simulink model "RL_TTS3_Controller_Blank"  (R2019b)
settings: Solver=FixedStepAuto  StartTime=0.0  StopTime=10.0  FixedStep=0.01  RelTol=1e-3
PostLoadFcn:
  | if any(exist('dsrtsu_mdlpostloadfcn', 'file') ~= 0), dsrtsu_mdlpostloadfcn('Execute', bdroot); end
values from neighbouring files (symbols this model uses):
  SetPumpR = 0    [RL_TTS3_Controller_Blank.mat]    (also in RL_TTS3_Controller_Blank_DefaultVal.mat)
  ValveLD_close = 0    [RL_TTS3_Controller_Blank.mat]    (also in RL_TTS3_Controller_Blank_DefaultVal.mat)
  ValveLD_open = 0    [RL_TTS3_Controller_Blank.mat]    (also in RL_TTS3_Controller_Blank_DefaultVal.mat)
  ValveLM_close = 0    [RL_TTS3_Controller_Blank.mat]    (also in RL_TTS3_Controller_Blank_DefaultVal.mat)
  ValveLM_open = 0    [RL_TTS3_Controller_Blank.mat]    (also in RL_TTS3_Controller_Blank_DefaultVal.mat)
  ValveMD_close = 0    [RL_TTS3_Controller_Blank.mat]    (also in RL_TTS3_Controller_Blank_DefaultVal.mat)
  ValveMD_open = 0    [RL_TTS3_Controller_Blank.mat]    (also in RL_TTS3_Controller_Blank_DefaultVal.mat)
  ValveMR_close = 0    [RL_TTS3_Controller_Blank.mat]    (also in RL_TTS3_Controller_Blank_DefaultVal.mat)
  ValveMR_open = 0    [RL_TTS3_Controller_Blank.mat]    (also in RL_TTS3_Controller_Blank_DefaultVal.mat)
  ValveRD_close = 0    [RL_TTS3_Controller_Blank.mat]    (also in RL_TTS3_Controller_Blank_DefaultVal.mat)
  ValveRD_open = 0    [RL_TTS3_Controller_Blank.mat]    (also in RL_TTS3_Controller_Blank_DefaultVal.mat)
libraries: simulink x1
settings Model: DSRTSU_INTERNAL_RTI_VER=550  DSRTSU_INTERNAL_RTI_TYPE=rti1104  RTICANMMDATA=struct('GeneralSetupData',struct('modelroot','E:\Will\RemoteLabs\TTS3\HostPC','generalsettings',struct('filesettings',struct('destfolder',struct('Name','RTICANMM_FILES','Check',1),'buildfolder',struct('Name','.','Check',1),'AbsDestfolder',struct('Name','E:\Will\RemoteLabs\TTS3\HostPC\RTICANMM_FILES'),'AbsBuildfolder',struct('Name','E:\Will\RemoteLabs\TTS3\HostPC'))),'options',struct('addpaths',1,'rmpaths',1,'addtrcexclusion',true,'cannavigator',struct('checkmonitoring',0),'show_usrtrc',0,'use_usrtrc',0),'advanced',struct('options',ones(1,100)),'MPSetup',{{}},'RTI',struct('Type','RTI1104','Ver','7.13','Date','02-Nov-2019'),'modelname','TTS3_Controller_Test_OL','block','TTS3_Controller_Test_OL'))  DSRTSU_INTERNAL_RTIFPGA=150  Creator=whendrix  LastModifiedBy=maxva
settings OptimizationCC: BlockReduction=off  OptimizeBlockIOStorage=off  BufferReuse=off  GlobalBufferReuse=off  ExpressionFolding=off  LocalBlockOutputs=off  OptimizeDataStoreBuffers=off  BusAssignmentInplaceUpdate=off
settings DebuggingCC: BusObjectLabelMismatch=none
settings HardwareCC: ProdBitPerPointer=32  ProdBitPerSizeT=32  ProdBitPerPtrDiffT=32  ProdLargestAtomicInteger=Integer  ProdEndianess=BigEndian  ProdWordSize=32  ProdHWDeviceType=Custom Processor->Custom  TargetIntDivRoundTo=Zero  TargetEndianess=BigEndian  TargetHWDeviceType=Custom Processor->Custom
settings ModelReferenceCC: ModelReferenceNumInstancesAllowed=Single  ModelReferenceMinAlgLoopOccurrences=on
settings SFSimCC: MATLABDynamicMemAlloc=off  CustomCodeUndefinedFunction=UseInterfaceOnly
settings RTWCC: Description=dSPACE DS1104 Hardware Platform  SystemTargetFile=rti1104.tlc  MakeCommand=make_rti  TemplateMakefile=rti1104.tmf
settings CodeAppCC: MaxIdLength=63
settings STFCustomTargetCC: ParMdlRefBuildCompliant=on  SystemTargetFile=rti1104.tlc
settings GRTTargetCC: TargetLangStandard=C89/C90 (ANSI)  CompOptLevelCompliant=off  ConcurrentExecutionCompliant=off  CombineOutputUpdateFcns=off  MatFileLogging=off  CPPClassGenCompliant=off  UseToolchainInfoCompliant=off

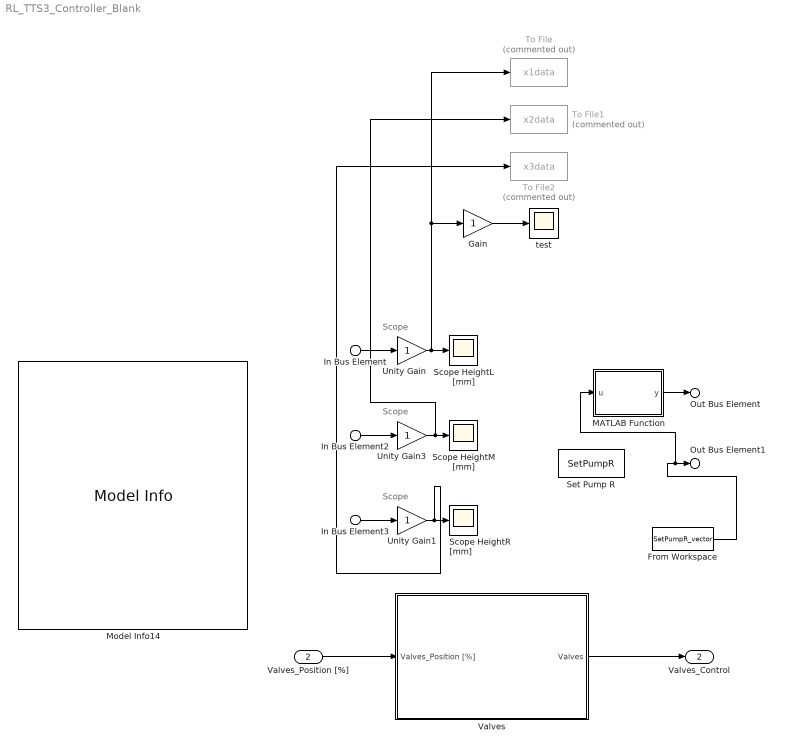
== system RL_TTS3_Controller_Blank ==
  note: Scope
  note: Scope
  note: Scope
  In Bus Element : Inport  PortName=Heights [mm]  Element=Left
  In Bus Element2 : Inport  PortName=Heights [mm]  Element=Middle
  In Bus Element3 : Inport  PortName=Heights [mm]  Element=Right
  Valves_Position [%] : Inport  Port=2  OutDataTypeStr=Bus: ValvesSOCI
  From Workspace : FromWorkspace  VariableName=SetPumpR_vector
  Gain : Gain
  MATLAB Function : MATLAB Function  TreatAsAtomicUnit=on
  Model Info14 : simulink/Model-Wide Utilities/Model Info  Frame=on  DisplayStringWithTags=|  HorizontalTextAlignment=Left  LeftAlignmentValue=0.02
      | Start model for the "Three Tank"
      | experiment on the "Three Tank" setup.
      | Version: 1.0
      | 
      | 
      | INFORMATION
      | ----------------------
      | 
      | Unity Gain block before Scope is needed for
      | RemoteLabs compatebility. 
      | Do not modify or remove!
      | 
      | Pump range:
      | 0 to 0.102 [l/s]
      | 
      | The 5 Valves are labeled according 
      | to their position:
      | 
      |    LM  MR
      |      X     X
      |  X      X      X
      | LD    MD   RD
      | 
      | L = Left
      | M = Middle
      | R = Right
      | D = Down
  Scope HeightL [mm] : Scope
  Scope HeightM [mm] : Scope
  Scope HeightR [mm] : Scope
  Set Pump R : Constant  Value=SetPumpR
  To File : ToFile  Commented=on  Filename=x1data  MatrixName=x1
  To File1 : ToFile  Commented=on  Filename=x2data  MatrixName=x2
  To File2 : ToFile  Commented=on  Filename=x3data  MatrixName=x3
  Unity Gain : Gain
  Unity Gain1 : Gain
  Unity Gain3 : Gain
  Valves : Subsystem  TreatAsAtomicUnit=on
  test : Scope
  Out Bus Element : Outport  VectorParamsAs1DForOutWhenUnconnected=off  PortName=Pumps [l/s]  Element=Left
  Out Bus Element1 : Outport  VectorParamsAs1DForOutWhenUnconnected=off  PortName=Pumps [l/s]  Element=Right
  Valves_Control : Outport  Port=2  OutDataTypeStr=Bus: ValvesSICO  VectorParamsAs1DForOutWhenUnconnected=off
  wires:
  Unity Gain3/1 -> To File1/1, Scope HeightM [mm]/1
  Unity Gain1/1 -> To File2/1, Scope HeightR [mm]/1
  In Bus Element/1 -> Unity Gain/1
  In Bus Element2/1 -> Unity Gain3/1
  In Bus Element3/1 -> Unity Gain1/1
  Valves/1(Valves) -> Valves_Control/1
  Valves_Position [%]/1 -> Valves/1(Valves_Position [%])
  Unity Gain/1 -> Gain/1, To File/1, Scope HeightL [mm]/1
  From Workspace/1 -> MATLAB Function/1(u), Out Bus Element1/1
  Gain/1 -> test/1
  MATLAB Function/1(y) -> Out Bus Element/1

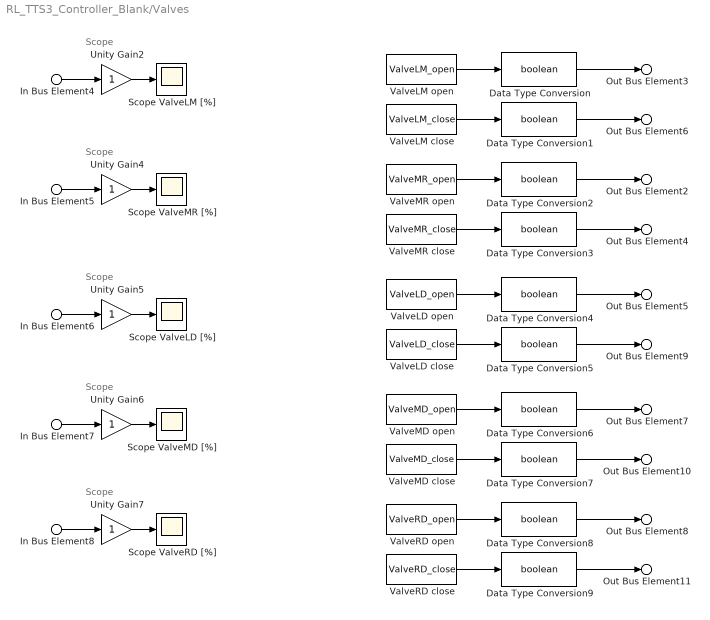
== system RL_TTS3_Controller_Blank/Valves ==
  note: Scope
  note: Scope
  note: Scope
  note: Scope
  note: Scope
  In Bus Element4 : Inport  PortName=Valves_Position [%]  Element=LeftMiddle
  In Bus Element5 : Inport  PortName=Valves_Position [%]  Element=MiddleRight
  In Bus Element6 : Inport  PortName=Valves_Position [%]  Element=LeftDown
  In Bus Element7 : Inport  PortName=Valves_Position [%]  Element=MiddleDown
  In Bus Element8 : Inport  PortName=Valves_Position [%]  Element=RightDown
  Data Type Conversion{,1..9} (10 alike) : DataTypeConversion  OutDataTypeStr=boolean
  Scope ValveLD [%] : Scope
  Scope ValveLM [%] : Scope
  Scope ValveMD [%] : Scope
  Scope ValveMR [%] : Scope
  Scope ValveRD [%] : Scope
  Unity Gain{2,4..7} (5 alike) : Gain
  ValveLD close : Constant  Value=ValveLD_close  OutDataTypeStr=double
  ValveLD open : Constant  Value=ValveLD_open  OutDataTypeStr=double
  ValveLM close : Constant  Value=ValveLM_close  OutDataTypeStr=double
  ValveLM open : Constant  Value=ValveLM_open  OutDataTypeStr=double
  ValveMD close : Constant  Value=ValveMD_close  OutDataTypeStr=double
  ValveMD open : Constant  Value=ValveMD_open  OutDataTypeStr=double
  ValveMR close : Constant  Value=ValveMR_close  OutDataTypeStr=double
  ValveMR open : Constant  Value=ValveMR_open  OutDataTypeStr=double
  ValveRD close : Constant  Value=ValveRD_close  OutDataTypeStr=double
  ValveRD open : Constant  Value=ValveRD_open  OutDataTypeStr=double
  Out Bus Element8 : Outport  VectorParamsAs1DForOutWhenUnconnected=off  PortName=Valves  Element=RightDown.Open
  Out Bus Element11 : Outport  VectorParamsAs1DForOutWhenUnconnected=off  PortName=Valves  Element=RightDown.Close
  Out Bus Element5 : Outport  VectorParamsAs1DForOutWhenUnconnected=off  PortName=Valves  Element=LeftDown.Open
  Out Bus Element9 : Outport  VectorParamsAs1DForOutWhenUnconnected=off  PortName=Valves  Element=LeftDown.Close
  Out Bus Element7 : Outport  VectorParamsAs1DForOutWhenUnconnected=off  PortName=Valves  Element=MiddleDown.Open
  Out Bus Element10 : Outport  VectorParamsAs1DForOutWhenUnconnected=off  PortName=Valves  Element=MiddleDown.Close
  Out Bus Element2 : Outport  VectorParamsAs1DForOutWhenUnconnected=off  PortName=Valves  Element=MiddleRight.Open
  Out Bus Element4 : Outport  VectorParamsAs1DForOutWhenUnconnected=off  PortName=Valves  Element=MiddleRight.Close
  Out Bus Element3 : Outport  VectorParamsAs1DForOutWhenUnconnected=off  PortName=Valves  Element=LeftMiddle.Open
  Out Bus Element6 : Outport  VectorParamsAs1DForOutWhenUnconnected=off  PortName=Valves  Element=LeftMiddle.Close
  wires:
  In Bus Element5/1 -> Unity Gain4/1
  In Bus Element4/1 -> Unity Gain2/1
  In Bus Element7/1 -> Unity Gain6/1
  Unity Gain6/1 -> Scope ValveMD [%]/1
  In Bus Element6/1 -> Unity Gain5/1
  In Bus Element8/1 -> Unity Gain7/1
  Unity Gain7/1 -> Scope ValveRD [%]/1
  Unity Gain4/1 -> Scope ValveMR [%]/1
  Unity Gain5/1 -> Scope ValveLD [%]/1
  Unity Gain2/1 -> Scope ValveLM [%]/1
  ValveLM open/1 -> Data Type Conversion/1
  ValveRD open/1 -> Data Type Conversion8/1
  ValveMR close/1 -> Data Type Conversion3/1
  ValveLD open/1 -> Data Type Conversion4/1
  ValveMD close/1 -> Data Type Conversion7/1
  ValveMR open/1 -> Data Type Conversion2/1
  ValveRD close/1 -> Data Type Conversion9/1
  ValveLM close/1 -> Data Type Conversion1/1
  ValveMD open/1 -> Data Type Conversion6/1
  ValveLD close/1 -> Data Type Conversion5/1
  Data Type Conversion/1 -> Out Bus Element3/1
  Data Type Conversion1/1 -> Out Bus Element6/1
  Data Type Conversion2/1 -> Out Bus Element2/1
  Data Type Conversion3/1 -> Out Bus Element4/1
  Data Type Conversion4/1 -> Out Bus Element5/1
  Data Type Conversion5/1 -> Out Bus Element9/1
  Data Type Conversion6/1 -> Out Bus Element7/1
  Data Type Conversion7/1 -> Out Bus Element10/1
  Data Type Conversion8/1 -> Out Bus Element8/1
  Data Type Conversion9/1 -> Out Bus Element11/1

== matlab function RL_TTS3_Controller_Blank/MATLAB Function ==
  data: u input; y output
function y = fcn(u)
% 
Atank =1;
Dvalve = 1;
v4 = 1;
v5 = 1;
q = 5;
m = 4;
y=0;
BmCT = [0.001/Atank 0 0 0;
        0 0.001/Atank 0 0;
        0 0 0 0 ;
        0 0 0.01*v4*Dvalve 0;
        0 0 0 0.01*v5*Dvalve];
Cm = eye(5);
Dm = zeros(q,m);
Am = zeros(5,5);
Bm = zeros(5,4);
AmCT = eye(5);

coder.extrinsic('ss');
coder.extrinsic('c2d');
coder.extrinsic('ssdata');
coder.extrinsic('ctrb');
coder.extrinsic('dlqr');
coder.extrinsic('quadprog');
% [Am,Bm,~,~] = ssdata(c2d(ss(AmCT,BmCT,Cm,Dm),Ts));
y = 0.75*u;
